simulink model "IAE"  (R2018a)
settings: Solver=VariableStepAuto  StartTime=0.0  StopTime=150  RelTol=1e-3
values from neighbouring files (symbols this model uses):
  k = 9.22    [Controlador2GDL.m]    (also in ControladorAlfaroPI1GDL_ControlEstricto.m; ControladorAlfaroPI1GDL_ControlSuave.m; Examen2.m)
  L = 3.17    [Controlador2GDL.m]    (also in ControladorAlfaroPI1GDL_ControlEstricto.m; ControladorAlfaroPI1GDL_ControlSuave.m; Examen2.m)
  T = 34.31    [Controlador2GDL.m]    (also in ControladorAlfaroPI1GDL_ControlEstricto.m; ControladorAlfaroPI1GDL_ControlSuave.m; Examen2.m)
  Ts = 0.1    [Examen2.m]
libraries: simulink x2
settings Model: Creator=wivill  LastModifiedBy=wivill

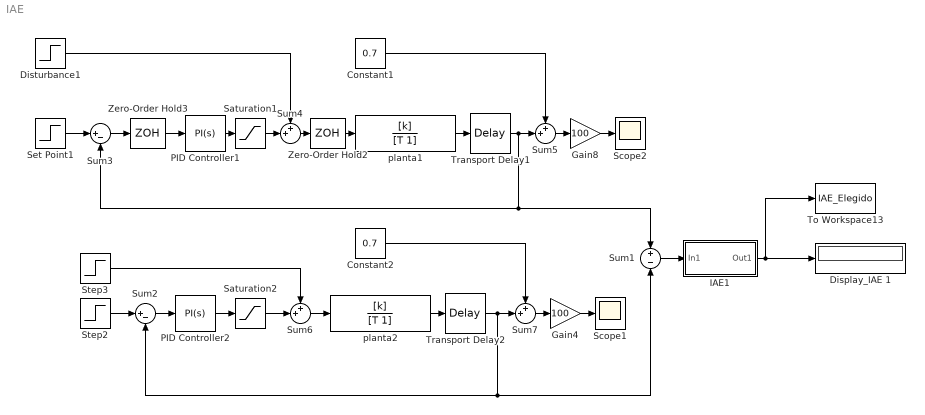
== system IAE ==
  Constant1 : Constant  Value=0.7
  Constant2 : Constant  Value=0.7
  Display_IAE 1 : Display
  Disturbance1 : Step  Time=30  After=-0.05  SampleTime=0
  Gain4 : Gain  Gain=100
  Gain8 : Gain  Gain=100
  IAE1 : Subsystem
      mask help:
      | IAE performacne index
      |
      | output = int |input| dt
      mask Display:
      | disp('IAE')
      | port_label('input',1,'e')
      | port_label('output',1,'iae')
  PID Controller1 : simulink/Continuous/PID Controller  Controller=PI  TimeDomain=Continuous-time  SampleTime=-1  IntegratorMethod=Forward Euler  FilterMethod=Forward Euler  Form=Ideal  UseFilter=on  ControllerParametersSource=internal  P=(0.57*T)/(k*L)  I=1/(T)  D=0  N=100  InitialConditionSource=internal  InitialConditionForIntegrator=0  InitialConditionForFilter=0  ExternalReset=none  LimitOutput=off  UpperSaturationLimit=inf  LowerSaturationLimit=-inf  LinearizeAsGain=on  AntiWindupMode=none  Kb=1  TrackingMode=off  Kt=1  PParamMin=[]  PParamMax=[]  IParamMin=[]  IParamMax=[]  DParamMin=[]  DParamMax=[]  NParamMin=[]  NParamMax=[]  KbParamMin=[]  KbParamMax=[]  KtParamMin=[]  KtParamMax=[]  POutMin=[]  POutMax=[]  IOutMin=[]  IOutMax=[]  DOutMin=[]  DOutMax=[]  NOutMin=[]  NOutMax=[]  KbOutMin=[]  KbOutMax=[]  KtOutMin=[]  KtOutMax=[]  IntegratorOutMin=[]  IntegratorOutMax=[]  FilterOutMin=[]  FilterOutMax=[]  SumOutMin=[]  SumOutMax=[]  SumI1OutMin=[]  SumI1OutMax=[]  SumI2OutMin=[]  SumI2OutMax=[]  SumI3OutMin=[]  SumI3OutMax=[]  SumDOutMin=[]  SumDOutMax=[]  SaturationOutMin=[]  SaturationOutMax=[]  IntegratorContinuousStateAttributes=''  IntegratorStateMustResolveToSignalObject=off  IntegratorRTWStateStorageClass=Auto  FilterContinuousStateAttributes=''  FilterStateMustResolveToSignalObject=off  FilterRTWStateStorageClass=Auto  DifferentiatorICPrevScaledInput=0  DifferentiatorOutMin=[]  DifferentiatorOutMax=[]  InitialConditionSetting=State (most efficient)  FilterDiffOutCoefMin=[]  FilterDiffOutCoefMax=[]  SumDenOutMin=[]  SumDenOutMax=[]  SumNumOutMin=[]  SumNumOutMax=[]  ReciprocalOutMin=[]  ReciprocalOutMax=[]  DivideOutMin=[]  DivideOutMax=[]  TunerSelectOption=Transfer Function Based (PID Tuner App)
  PID Controller2 : simulink/Continuous/PID Controller  Controller=PI  TimeDomain=Continuous-time  SampleTime=-1  IntegratorMethod=Forward Euler  FilterMethod=Forward Euler  Form=Ideal  UseFilter=on  ControllerParametersSource=internal  P=(0.57*T)/(k*L)  I=1/(T)  D=0  N=100  InitialConditionSource=internal  InitialConditionForIntegrator=0  InitialConditionForFilter=0  ExternalReset=none  LimitOutput=off  UpperSaturationLimit=inf  LowerSaturationLimit=-inf  LinearizeAsGain=on  AntiWindupMode=none  Kb=1  TrackingMode=off  Kt=1  PParamMin=[]  PParamMax=[]  IParamMin=[]  IParamMax=[]  DParamMin=[]  DParamMax=[]  NParamMin=[]  NParamMax=[]  KbParamMin=[]  KbParamMax=[]  KtParamMin=[]  KtParamMax=[]  POutMin=[]  POutMax=[]  IOutMin=[]  IOutMax=[]  DOutMin=[]  DOutMax=[]  NOutMin=[]  NOutMax=[]  KbOutMin=[]  KbOutMax=[]  KtOutMin=[]  KtOutMax=[]  IntegratorOutMin=[]  IntegratorOutMax=[]  FilterOutMin=[]  FilterOutMax=[]  SumOutMin=[]  SumOutMax=[]  SumI1OutMin=[]  SumI1OutMax=[]  SumI2OutMin=[]  SumI2OutMax=[]  SumI3OutMin=[]  SumI3OutMax=[]  SumDOutMin=[]  SumDOutMax=[]  SaturationOutMin=[]  SaturationOutMax=[]  IntegratorContinuousStateAttributes=''  IntegratorStateMustResolveToSignalObject=off  IntegratorRTWStateStorageClass=Auto  FilterContinuousStateAttributes=''  FilterStateMustResolveToSignalObject=off  FilterRTWStateStorageClass=Auto  DifferentiatorICPrevScaledInput=0  DifferentiatorOutMin=[]  DifferentiatorOutMax=[]  InitialConditionSetting=State (most efficient)  FilterDiffOutCoefMin=[]  FilterDiffOutCoefMax=[]  SumDenOutMin=[]  SumDenOutMax=[]  SumNumOutMin=[]  SumNumOutMax=[]  ReciprocalOutMin=[]  ReciprocalOutMax=[]  DivideOutMin=[]  DivideOutMax=[]  TunerSelectOption=Transfer Function Based (PID Tuner App)
  Saturation1 : Saturate  UpperLimit=1  LowerLimit=-0.1
  Saturation2 : Saturate  UpperLimit=1  LowerLimit=-0.1
  Scope1 : Scope
  Scope2 : Scope
  Set Point1 : Step  Time=0  After=0.1  SampleTime=0
  Step2 : Step  Time=0  After=0.1  SampleTime=0
  Step3 : Step  Time=30  After=-0.05  SampleTime=0
  Sum1 : Sum  Inputs=+|-
  Sum2 : Sum  Inputs=|+-
  Sum3 : Sum  Inputs=|+-
  Sum{4..7} (4 alike) : Sum  Inputs=++|
  To Workspace13 : ToWorkspace  VariableName=IAE_Elegido  SaveFormat=Timeseries  SampleTime=Ts
  Transport Delay1 : TransportDelay  DelayTime=L
  Transport Delay2 : TransportDelay  DelayTime=L
  Zero-Order Hold2 : ZeroOrderHold  SampleTime=Ts
  Zero-Order Hold3 : ZeroOrderHold  SampleTime=Ts
  planta1 : TransferFcn  Numerator=[k]  Denominator=[T 1]  ContinuousStateAttributes='planta'
  planta2 : TransferFcn  Numerator=[k]  Denominator=[T 1]  ContinuousStateAttributes='planta'
  wires:
  Constant1/1 -> Sum5/1
  Gain8/1 -> Scope2/1
  Sum5/1 -> Gain8/1
  Zero-Order Hold2/1 -> planta1/1
  Sum3/1 -> Zero-Order Hold3/1
  Disturbance1/1 -> Sum4/1
  Saturation1/1 -> Sum4/2
  Sum4/1 -> Zero-Order Hold2/1
  planta1/1 -> Transport Delay1/1
  Set Point1/1 -> Sum3/1
  Transport Delay1/1 -> Sum5/2, Sum1/1, Sum3/2
  PID Controller1/1 -> Saturation1/1
  Zero-Order Hold3/1 -> PID Controller1/1
  Step2/1 -> Sum2/1
  Step3/1 -> Sum6/1
  Sum2/1 -> PID Controller2/1
  Constant2/1 -> Sum7/1
  Saturation2/1 -> Sum6/2
  PID Controller2/1 -> Saturation2/1
  Transport Delay2/1 -> Sum7/2, Sum1/2, Sum2/2
  Gain4/1 -> Scope1/1
  planta2/1 -> Transport Delay2/1
  Sum6/1 -> planta2/1
  Sum7/1 -> Gain4/1
  IAE1/1(Out1) -> To Workspace13/1, Display_IAE 1/1
  Sum1/1 -> IAE1/1(In1)

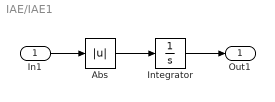
== system IAE/IAE1 ==
  In1 : Inport
  Abs : Abs
  Integrator : Integrator
  Out1 : Outport
  wires:
  In1/1 -> Abs/1
  Integrator/1 -> Out1/1
  Abs/1 -> Integrator/1
